simulink model "model"  (R2017b)
settings: Solver=VariableStepAuto  StartTime=0.0  StopTime=300  RelTol=1e-3
values from neighbouring files (symbols this model uses):
  A = [(-su*(g/(sqrt((2/rho)*(kc*(u_0-u_N)^2 - rho*g*(x_1_0+offset1)))))-(v_T_0*st)*(g/(sqrt(2*g*(x_1_0-x_2_0))))) ((v_T_0*st)*(g/(sqrt(2*g*(x_1_0-x_2_0))))) ... (first row only)    [main_opo.m]
  B = [su*(2/rho * kc *(u_0 - u_N))/(sqrt(2/rho * (kc * (u_0 - u_N)^2 - rho * g * (x_1_0 - offset1)))) -st * sqrt(2*g*(x_1_0 - x_2_0)) 0 ... (first row only)    [main_opo.m]
  C = eye(2)    [main_opo.m]
  D = zeros(2,3)    [main_opo.m]
  kc = (1000*9.81*(0.5344+offset1))/(0.55-u_N)^2    (= 25577.3756062)    [main_opo.m]
  offset1 = 0.07637    [main_opo.m]
  offset2 = -0.06864    [main_opo.m]
  prac_in = [u_0; v_T_0; v_o_0]    [main_opo.m]
  prac_out = [x_1_0;x_2_0]    [main_opo.m]
  so = 1.1*sqrt(2*ho/g)/to    [main_opo.m]
  su = 1.1*sqrt(2*hu/g)/tu    [main_opo.m]
libraries: dsppolyfun x1
settings Model: Creator=repro  LastModifiedBy=repro

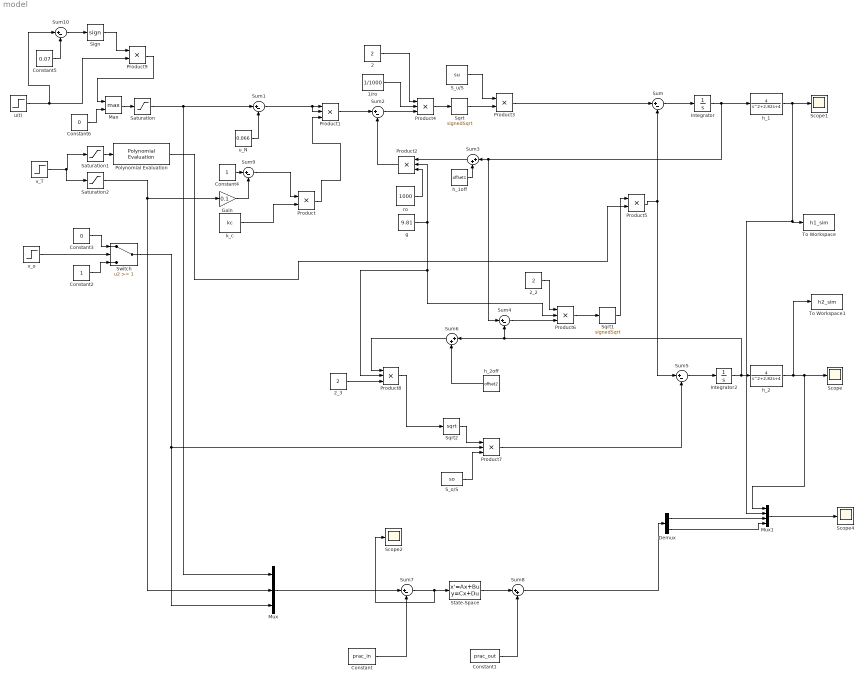
== system model ==
  "1/ro " : Constant  Value=1/1000
  "2 " : Constant  Value=2
  "2_2 " : Constant  Value=2
  "2_3 " : Constant  Value=2
  Constant : Constant  Value=prac_in
  Constant1 : Constant  Value=prac_out
  Constant2 : Constant
  Constant3 : Constant  Value=0
  Constant4 : Constant
  Constant5 : Constant  Value=0.07
  Constant6 : Constant  Value=0
  Demux : Demux  Outputs=2
  Gain : Gain  Gain=0.1
  Integrator : Integrator  InitialCondition=0.03  LimitOutput=on  UpperSaturationLimit=1  LowerSaturationLimit=0.03
  Integrator2 : Integrator  InitialCondition=0.07  LimitOutput=on  UpperSaturationLimit=1  LowerSaturationLimit=0.07
  Max : MinMax  Function=max  Inputs=2
  Mux : Mux  Inputs=3
  Mux1 : Mux
  Polynomial Evaluation : dsppolyfun/Polynomial Evaluation  useConstCoeffs=on  constCoeffs=p
      settings: SourceProductName=DSP System Toolbox  SourceProductBaseCode=DS
  Product{,3,5,9} (4 alike) : Product
  Product{1..2,4,6..8} (6 alike) : Product  Inputs=3
  S_o/S : Constant  Value=so
  "S_u/S " : Constant  Value=su
  Saturation : Saturate  UpperLimit=1  LowerLimit=0
  Saturation1 : Saturate  UpperLimit=1  LowerLimit=0.31
  Saturation2 : Saturate  UpperLimit=1  LowerLimit=0
  Scope{,1..2,4} (4 alike) : Scope
  Sign : Signum
  Sqrt : Sqrt  Operator=signedSqrt  SaturateOnIntegerOverflow=on
  Sqrt1 : Sqrt  Operator=signedSqrt  SaturateOnIntegerOverflow=on
  Sqrt2 : Sqrt  SaturateOnIntegerOverflow=on
  State-Space : StateSpace  A=A  B=B  C=C  D=D  InitialCondition=0
  Sum{,1..2,4..5,7,9..10} (8 alike) : Sum  Inputs=|+-
  Sum3 : Sum  Inputs=|++
  Sum6 : Sum  Inputs=|++
  Sum8 : Sum  Inputs=|++
  Switch : Switch  Threshold=1
  To Workspace : ToWorkspace  VariableName=h1_sim  SaveFormat=Timeseries  SampleTime=-1
  To Workspace1 : ToWorkspace  VariableName=h2_sim  SaveFormat=Timeseries  SampleTime=-1
  g : Constant  Value=9.81
  "h_1 " : TransferFcn  Numerator=[4]  Denominator=[1 2.82 4]
  h_1off : Constant  Value=offset1
  h_2 : TransferFcn  Numerator=[4]  Denominator=[1 2.82 4]
  h_2off : Constant  Value=offset2
  k_c : Constant  Value=kc
  ro : Constant  Value=1000
  u(t) : Step  Time=100  Before=0.55  After=0.6  SampleTime=0
  u_N : Constant  Value=0.066
  v_T : Step  Time=0  After=0.5  SampleTime=0
  v_o : Step  Time=0  SampleTime=0
  wires:
  Sum/1 -> Integrator/1
  u_N/1 -> Sum1/2
  Sum1/1 -> Product1/2, Product1/1
  Product1/1 -> Sum2/1
  Integrator/1 -> Sum4/1, Sum3/1, "h_1 "/1
  h_1off/1 -> Sum3/2
  Product2/1 -> Sum2/2
  Sum3/1 -> Product2/1
  ro/1 -> Product2/3
  g/1 -> Product6/2, Product8/2, Product2/2
  "2 "/1 -> Product4/1
  "1/ro "/1 -> Product4/2
  Sum2/1 -> Product4/3
  Product4/1 -> Sqrt/1
  Product3/1 -> Sum/1
  Integrator2/1 -> Sum4/2, Sum6/1, h_2/1
  "2_2 "/1 -> Product6/1
  Sum4/1 -> Product6/3
  Product6/1 -> Sqrt1/1
  Product5/1 -> Sum5/1, Sum/2
  Sqrt2/1 -> Product7/1
  Product7/1 -> Sum5/2
  Product8/1 -> Sqrt2/1
  "2_3 "/1 -> Product8/3
  Sum6/1 -> Product8/1
  h_2off/1 -> Sum6/2
  Sum5/1 -> Integrator2/1
  "h_1 "/1 -> Mux1/2, To Workspace/1, Scope1/1
  h_2/1 -> Mux1/1, Scope/1, To Workspace1/1
  Saturation/1 -> Mux/1, Sum1/1
  Sqrt/1 -> Product3/2
  "S_u/S "/1 -> Product3/1
  S_o/S/1 -> Product7/3
  Product/1 -> Product1/3
  Constant1/1 -> Sum8/2
  Constant/1 -> Sum7/2
  Sum7/1 -> Scope2/1, State-Space/1
  State-Space/1 -> Sum8/1
  Mux/1 -> Sum7/1
  Switch/1 -> Mux/3, Product7/2
  Sum8/1 -> Demux/1
  Mux1/1 -> Scope4/1
  v_o/1 -> Switch/2
  Constant2/1 -> Switch/3
  Constant3/1 -> Switch/1
  Saturation1/1 -> Polynomial Evaluation/1
  v_T/1 -> Saturation2/1, Saturation1/1
  Saturation2/1 -> Mux/2, Gain/1
  Constant4/1 -> Sum9/1
  Gain/1 -> Sum9/2
  Sum9/1 -> Product/1
  Sqrt1/1 -> Product5/1
  k_c/1 -> Product/2
  Max/1 -> Saturation/1
  Sum10/1 -> Sign/1
  Constant5/1 -> Sum10/2
  u(t)/1 -> Product9/2, Sum10/1
  Sign/1 -> Product9/1
  Product9/1 -> Max/1
  Constant6/1 -> Max/2
  Demux/1 -> Mux1/3
  Polynomial Evaluation/1 -> Product5/2
  Demux/2 -> Mux1/4
